simulink model "inductioncontrolsimnewest"  (R2015a)
settings: Solver=ode45  StartTime=0.0  StopTime=5  RelTol=1e-3
settings Model: Creator=kbmaj  LastModifiedBy=kbmaj

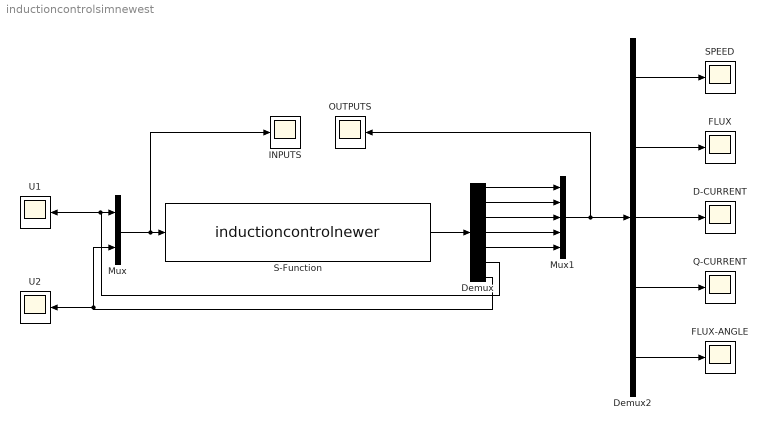
== system inductioncontrolsimnewest ==
  " FLUX-ANGLE" : Scope
      settings: TimeRange=5  YMin=2.675e+06  YMax=3.075e+06  SaveName=ScopeData6
  " Q-CURRENT" : Scope
      settings: YMin=9350  YMax=9465  SaveName=ScopeData5
  D-CURRENT : Scope
      settings: YMin=-6000  YMax=9000  SaveName=ScopeData4
  Demux : Demux  Outputs=7
  Demux2 : Demux  Outputs=5
  FLUX : Scope
      settings: YMin=-4.5  YMax=4.5  SaveName=ScopeData3
  INPUTS : Scope
      settings: YMin=-4.5e+08  YMax=5.5e+08
  Mux : Mux  Inputs=2
  Mux1 : Mux  Inputs=5
  OUTPUTS : Scope
      settings: YMin=-950000  YMax=200000  SaveName=ScopeData11
  S-Function : S-Function  FunctionName=inductioncontrolnewer
  SPEED : Scope
      settings: TimeRange=10  YMin=-12000  YMax=11000  SaveName=ScopeData2
  U1 : Scope
      settings: YMin=0  YMax=120000  SaveName=ScopeData9
  U2 : Scope
      settings: YMin=-2.25e+12  YMax=2.25e+12  SaveName=ScopeData10
  wires:
  Mux/1 -> S-Function/1, INPUTS/1
  Mux1/1 -> OUTPUTS/1, Demux2/1
  Demux2/1 -> SPEED/1
  Demux2/2 -> FLUX/1
  Demux2/3 -> D-CURRENT/1
  Demux2/4 -> " Q-CURRENT"/1
  Demux2/5 -> " FLUX-ANGLE"/1
  Demux/7 -> U2/1, Mux/2
  Demux/6 -> Mux/1, U1/1
  S-Function/1 -> Demux/1
  Demux/1 -> Mux1/1
  Demux/2 -> Mux1/2
  Demux/3 -> Mux1/3
  Demux/4 -> Mux1/4
  Demux/5 -> Mux1/5
